simulink model "EASTO_Simulink"  (R2022a)
settings: Solver=VariableStepAuto  StartTime=0.0  StopTime=100.0  RelTol=1e-3
settings Model: Creator=arkiven4  LastModifiedBy=arkiven4

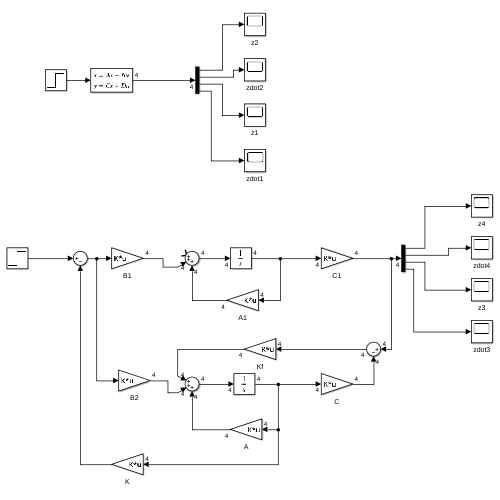
[thumbnail: Simulink's stored preview of the top-level diagram]
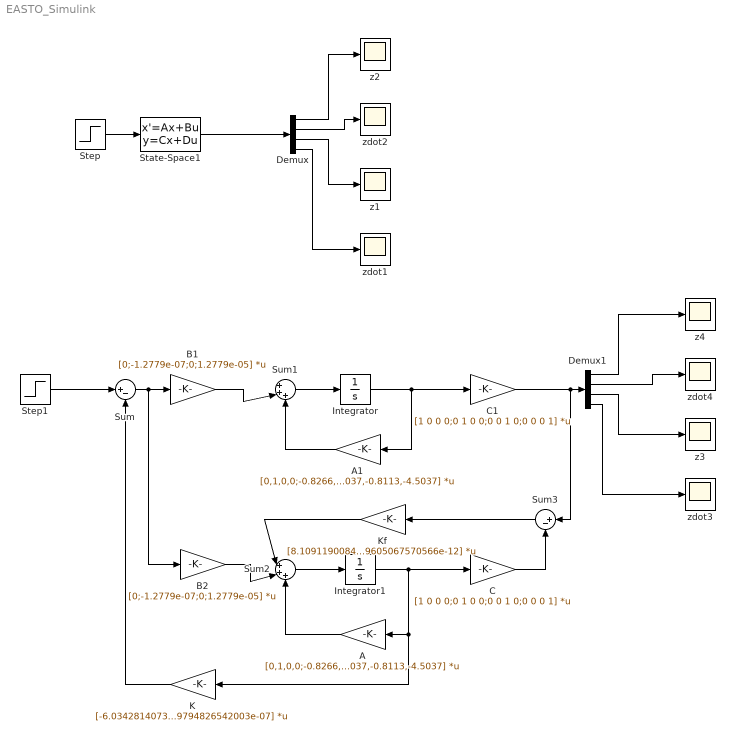
== system EASTO_Simulink ==
  A : Gain  Gain=[0,1,0,0;-0.8266,-0.4974,0.0081,0.0450;0,0,0,1;0.8113,4.5037,-0.8113,-4.5037]  Multiplication=Matrix(K*u)
  A1 : Gain  Gain=[0,1,0,0;-0.8266,-0.4974,0.0081,0.0450;0,0,0,1;0.8113,4.5037,-0.8113,-4.5037]  Multiplication=Matrix(K*u)
  B1 : Gain  Gain=[0;-1.2779e-07;0;1.2779e-05]  Multiplication=Matrix(K*u)
  B2 : Gain  Gain=[0;-1.2779e-07;0;1.2779e-05]  Multiplication=Matrix(K*u)
  C : Gain  Gain=[1 0 0 0;0 1 0 0;0 0 1 0;0 0 0 1]  Multiplication=Matrix(K*u)
  C1 : Gain  Gain=[1 0 0 0;0 1 0 0;0 0 1 0;0 0 0 1]  Multiplication=Matrix(K*u)
  Demux : Demux
  Demux1 : Demux
  Integrator : Integrator
  Integrator1 : Integrator
  K : Gain  Gain=[-6.03428140733562e-07,4.41695800719318e-07,7.87541077548334e-07,3.19794826542003e-07]  Multiplication=Matrix(K*u)
  Kf : Gain  Gain=[8.10911900849225e-17,-2.77610056424295e-18,2.69188143628669e-17,-3.60765248007911e-15;2.23664577705347e-18,2.28641981033545e-16,3.60756375299832e-15,-1.62763185263795e-14;4.25312178761283e-17,3.61207441423341e-15,2.23388036360143e-12,1.55979167168727e-18;-3.60358775540895e-15,-1.62846648577553e-14,1.97045813847738e-17,1.79605067570566e-12]  Multiplication=Matrix(K*u)
  State-Space1 : StateSpace  A=[0 1 0 0; -0.8266 -0.4974 0.0081 0.0450; 0 0 0 1; 0.8113 4.5037 -0.8113 -4.5037]  B=[0;-1.2779e-07;0;1.2779e-05]  C=[1 0 0 0;0 1 0 0;0 0 1 0;0 0 0 1]  D=[0;0;0;0]  InitialCondition=0
  Step : Step  SampleTime=0
  Step1 : Step  SampleTime=0
  Sum : Sum  Inputs=|+-
  Sum1 : Sum  Inputs=|+++
  Sum2 : Sum  Inputs=|+++
  Sum3 : Sum  Inputs=|+-
  z{1..4} (4 alike) : Scope
  zdot{1..4} (4 alike) : Scope
  wires:
  State-Space1/1 -> Demux/1
  Demux/1 -> z2/1
  Demux/2 -> zdot2/1
  Demux/3 -> z1/1
  Demux/4 -> zdot1/1
  Sum1/1 -> Integrator/1
  Step1/1 -> Sum/1
  Sum/1 -> B2/1, B1/1
  K/1 -> Sum/2
  B1/1 -> Sum1/2
  A1/1 -> Sum1/3
  Integrator/1 -> A1/1, C1/1
  Sum2/1 -> Integrator1/1
  C/1 -> Sum3/2
  C1/1 -> Sum3/1, Demux1/1
  Integrator1/1 -> K/1, A/1, C/1
  A/1 -> Sum2/3
  Sum3/1 -> Kf/1
  Demux1/1 -> z4/1
  Demux1/2 -> zdot4/1
  Demux1/3 -> z3/1
  Demux1/4 -> zdot3/1
  Step/1 -> State-Space1/1
  Kf/1 -> Sum2/1
  B2/1 -> Sum2/2
